simulink model "projekt3_sim"  (R2022b)
settings: Solver=VariableStepAuto  StartTime=0.0  StopTime=200  RelTol=1e-3
values from neighbouring files (symbols this model uses):
  ki = Y(i)    [projekt3.m]
  kp = X(i)    [projekt3.m]
  Ms = [1 4 1 -6]    [projekt3.m]
undefined symbols (not defined in the file or in its folder): Kp
settings Model: Creator=filip  LastModifiedBy=Lenovo

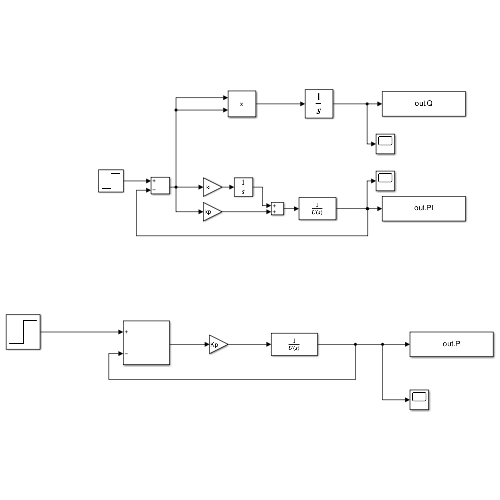
[thumbnail: Simulink's stored preview of the top-level diagram]
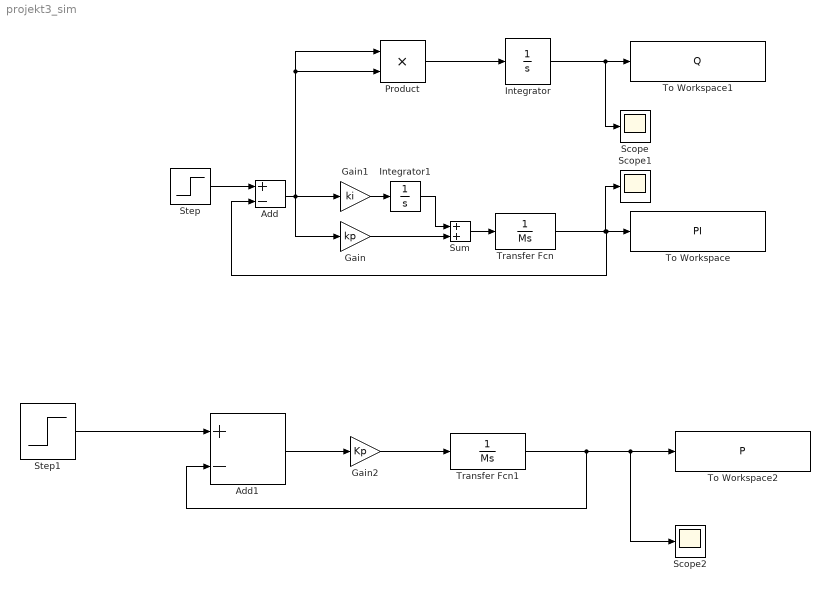
== system projekt3_sim ==
  Add : Sum  Inputs=+-
  Add1 : Sum  Inputs=+-
  Gain : Gain  Gain=kp
  Gain1 : Gain  Gain=ki
  Gain2 : Gain  Gain=Kp
  Integrator : Integrator
  Integrator1 : Integrator
  Product : Product
  Scope : Scope
  Scope1 : Scope
  Scope2 : Scope
  Step : Step  SampleTime=0
  Step1 : Step  SampleTime=0
  Sum : Sum  Inputs=+|+
  To Workspace : ToWorkspace  VariableName=PI  SampleTime=-1
  To Workspace1 : ToWorkspace  VariableName=Q  SampleTime=-1
  To Workspace2 : ToWorkspace  VariableName=P  SampleTime=-1
  Transfer Fcn : TransferFcn  Denominator=Ms
  Transfer Fcn1 : TransferFcn  Denominator=Ms
  wires:
  Step/1 -> Add/1
  Add/1 -> Product/2, Product/1, Gain1/1, Gain/1
  Transfer Fcn/1 -> To Workspace/1, Add/2, Scope1/1
  Integrator/1 -> To Workspace1/1, Scope/1
  Product/1 -> Integrator/1
  Gain1/1 -> Integrator1/1
  Gain2/1 -> Transfer Fcn1/1
  Add1/1 -> Gain2/1
  Step1/1 -> Add1/1
  Transfer Fcn1/1 -> Add1/2, Scope2/1, To Workspace2/1
  Sum/1 -> Transfer Fcn/1
  Integrator1/1 -> Sum/1
  Gain/1 -> Sum/2
